simulink model "demo3_model"  (R2024b)
settings: Solver=FixedStepAuto  StartTime=0.0  StopTime=5/60  FixedStep=1/12000  RelTol=1e-3
InitFcn:
  | Vdc1= 35;
  | Vdc2= 35;
  | Vdc3= 35;
  | Vdc4= 35;
  | Vdc5= 35;
  | 
  | GA_th = [58    21    17    49    14];
undefined symbols (not defined in the file): Vdc
libraries: spsDCVoltageSourceLib x5, spsFullBridgeConverterLib x5, spsVoltageMeasurementLib x5, spsSeriesRLCBranchLib x1, simulink x1, spspowerguiLib x1
settings Model: Creator=pgm
settings SolverCC: AlgebraicLoopSolver=TrustRegion
settings DataIOCC: ReturnWorkspaceOutputs=off
settings ModelReferenceCC: EnableRefExpFcnMdlSchedulingChecks=on
settings RTWCC: GPUComputeCapability=3.5

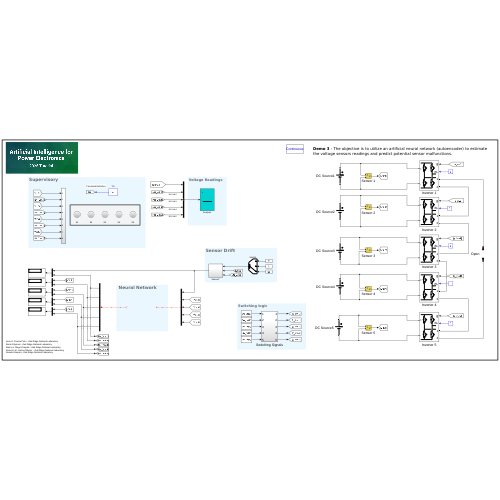
[thumbnail: Simulink's stored preview of the top-level diagram]
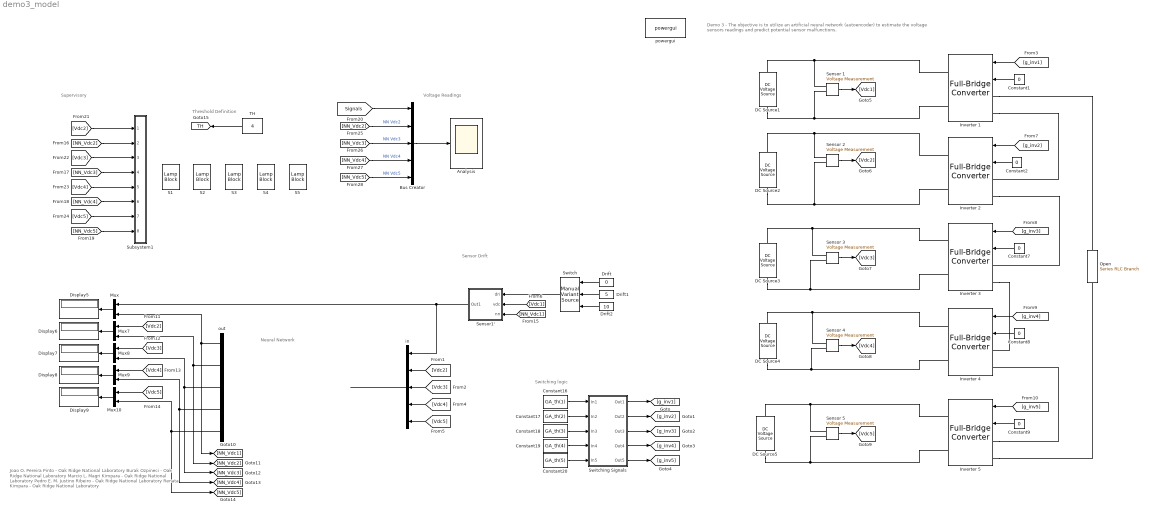
== system demo3_model ==
  note: Threshold Definition
  note: Switching logic
  note: Demo 3 - The objective is to utilize an artificial neural network (autoencoder) to estimate the voltage sensors readings and predict potential sensor malfunctions.
  note: Neural Network
  note: Sensor Drift
  note: Supervisory
  note: Voltage Readings
  note: Joao O. Pereira Pinto - Oak Ridge National Laboratory
      | Burak Ozpineci - Oak Ridge National Laboratory
      | Marcio L. Magri Kimpara - Oak Ridge National Laboratory
      | Pedro E. M. Justino Ribeiro - Oak Ridge National Laboratory
      | Renata Kimpara - Oak Ridge National Laboratory
  Analysis : Scope
  Bus Creator : BusCreator  Inputs=5
  Constant{1..2,7..9} (5 alike) : Constant  Value=0
  Constant16 : Constant  Value=GA_th(1)
  Constant17 : Constant  Value=GA_th(2)
  Constant18 : Constant  Value=GA_th(3)
  Constant19 : Constant  Value=GA_th(4)
  Constant20 : Constant  Value=GA_th(5)
  DC Source{1..5} (5 alike) : spsDCVoltageSourceLib/DC Voltage Source  Amplitude=Vdc  Measurements=None
  Display{5..9} (5 alike) : Display
  Drift : Constant  Value=0
  Drift1 : Constant  Value=5
  Drift2 : Constant  Value=10
  Inverter {1..5} (5 alike) : spsFullBridgeConverterLib/Full-Bridge Converter  ModelType=Switching devices  Ron=1e-3  Rs=1e6  Cs=inf  Vforward=[0,0]  Ron_Diode=1e-3  Rs_Diode=1e6  Cs_Diode=inf  Vf_Diode=1e-3  Rs_CurrentSource=inf  Ron_ACsource=1e-3
      settings: LibrarySourceBlock=sps_lib/Power Electronics/Full-Bridge Converter
  Mux{,7..10} (5 alike) : Mux  Inputs=2
  Open : spsSeriesRLCBranchLib/Series RLC Branch  LConnTagsString=__new0  RConnTagsString=__new0  BranchType=Open circuit  Resistance=10e3  Inductance=1e-6  SetiL0=off  InitialCurrent=0  Capacitance=400e-6  Setx0=off  InitialVoltage=0  Measurements=None
  S{1..5} (5 alike) : LampBlock  LabelPosition=Hide
  Sensor {1..5} (5 alike) : spsVoltageMeasurementLib/Voltage Measurement  Tag=PoWeRsYsTeMmEaSuReMeNt  PhasorSimulation=off  OutputType=Magnitude  PSBequivalent=0
  Sensor1' : Subsystem
  Subsystem1 : Subsystem
  Switch : simulink/Signal Routing/Manual Variant Source  NumChoices=3  LabelModeActiveChoice=V_3
  Switching Signals : Subsystem
  TH : Constant  Value=4
  in : Mux  Inputs=5
  out : Demux  Outputs=5
  powergui : spspowerguiLib/powergui  Priority=1  SimulationMode=Continuous  SampleTime=1e-6  frequency=60  Iterations=50  frequencyindice=0  Pbase=100e6  ErrMax=1e-4  UnitsV=kV  UnitsW=MW  buscounter=0  FunctionMessages=off  echomessages=off  EnableUseOfTLC=off  CurrentSourceSwitches=off  DisableSnubberDevices=off  DisableRonSwitches=off  DisableVfSwitches=off  DisplayEquations=off  AutomaticDiscreteSolvers=off  SolverType=Tustin/Backward Euler (TBE)  Interpol=off  ExternalGateDelay=off  methode=off  Ts=100  x0status=blocks  SPID=on  SwTol=0  HookPort=off  NonlinearTolerance=1e-4  nMaxIteration=100  ContinueOnMaxIteration=off  RestoreLinks=warning  ResistiveCurrentMeasurement=off  Frange=[0:2:500]  Ylog=off  Xlog=on  ShowGrid=off  save=off  variable=ZData  structure=0  ZoomFFT=off  StartTime=0.0  cycles=1  DisplayStyle=1  fundamental=60  FreqAxis=off  MaxFrequency=1000  frequencyindicesteady=1  RmsSteady=1  display=off
  tag scope: TH=global
  wires:
  Constant1/1 -> Inverter 1/2
  Constant2/1 -> Inverter 2/2
  [g_inv1] -> Inverter 1/1
  [g_inv2] -> Inverter 2/1
  [g_inv4] -> Inverter 4/1
  [g_inv3] -> Inverter 3/1
  Constant8/1 -> Inverter 4/2
  Constant7/1 -> Inverter 3/2
  Constant9/1 -> Inverter 5/2
  [g_inv5] -> Inverter 5/1
  Constant16/1 -> Switching Signals/1(In1)
  Constant17/1 -> Switching Signals/2(In2)
  Constant18/1 -> Switching Signals/3(In3)
  Constant19/1 -> Switching Signals/4(In4)
  Constant20/1 -> Switching Signals/5(In5)
  Switching Signals/1(Out1) -> [g_inv1]
  Switching Signals/2(Out2) -> [g_inv2]
  Switching Signals/3(Out3) -> [g_inv3]
  Switching Signals/4(Out4) -> [g_inv4]
  Switching Signals/5(Out5) -> [g_inv5]
  in/1 -> ?
  ? -> out/1
  Sensor 1/1 -> [Vdc1]
  Sensor 2/1 -> [Vdc2]
  Sensor 5/1 -> [Vdc5]
  Sensor 4/1 -> [Vdc4]
  Sensor 3/1 -> [Vdc3]
  [Vdc2] -> in/2
  [Vdc4] -> in/4
  [Vdc5] -> in/5
  Mux/1 -> Display5/1
  Mux7/1 -> Display6/1
  Mux8/1 -> Display7/1
  Mux9/1 -> Display8/1
  Mux10/1 -> Display9/1
  Switch/1 -> Sensor1'/1(dri)
  [Vdc1] -> Sensor1'/2(vdc)
  [Vdc2] -> Mux7/1
  [Vdc3] -> Mux8/1
  [Vdc4] -> Mux9/1
  [Vdc5] -> Mux10/1
  out/1 -> Mux/2, [NN_Vdc1]
  out/2 -> Mux7/2, [NN_Vdc2]
  out/3 -> [NN_Vdc3], Mux8/2
  out/4 -> [NN_Vdc4], Mux9/2
  out/5 -> [NN_Vdc5], Mux10/2
  [NN_Vdc1] -> Sensor1'/3(nn)
  [Vdc3] -> in/3
  [Signals] -> Bus Creator/1
  [NN_Vdc2] -> Bus Creator/2  "NN Vdc2"
  [NN_Vdc3] -> Bus Creator/3  "NN Vdc3"
  [NN_Vdc4] -> Bus Creator/4  "NN Vdc4"
  [NN_Vdc5] -> Bus Creator/5  "NN Vdc5"
  Bus Creator/1 -> Analysis/1
  Drift2/1 -> Switch/3
  [NN_Vdc5] -> Subsystem1/8(In10)
  [Vdc2] -> Subsystem1/1(In3)
  [NN_Vdc4] -> Subsystem1/6(In8)
  [Vdc5] -> Subsystem1/7(In9)
  [Vdc4] -> Subsystem1/5(In7)
  [Vdc3] -> Subsystem1/3(In5)
  [NN_Vdc2] -> Subsystem1/2(In4)
  [NN_Vdc3] -> Subsystem1/4(In6)
  Drift/1 -> Switch/1
  Drift1/1 -> Switch/2
  TH/1 -> [TH]
  Sensor1'/1(Out1) -> Mux/1, in/1
  connections:
  Sensor 1/LConn1 -- DC Source1/RConn1 -- Inverter 1/RConn1
  Sensor 1/LConn2 -- DC Source1/LConn1 -- Inverter 1/RConn2
  Inverter 2/RConn1 -- DC Source2/RConn1 -- Sensor 2/LConn1
  Sensor 2/LConn2 -- DC Source2/LConn1 -- Inverter 2/RConn2
  Inverter 5/LConn2 -- Open/RConn1
  Inverter 1/LConn1 -- Open/LConn1
  Sensor 4/LConn1 -- DC Source4/RConn1 -- Inverter 4/RConn1
  DC Source3/LConn1 -- Sensor 3/LConn2 -- Inverter 3/RConn2
  Sensor 4/LConn2 -- DC Source4/LConn1 -- Inverter 4/RConn2
  DC Source3/RConn1 -- Sensor 3/LConn1 -- Inverter 3/RConn1
  Sensor 5/LConn2 -- DC Source5/LConn1 -- Inverter 5/RConn2
  Sensor 5/LConn1 -- DC Source5/RConn1 -- Inverter 5/RConn1
  Inverter 1/LConn2 -- Inverter 2/LConn1
  Inverter 2/LConn2 -- Inverter 3/LConn1
  Inverter 3/LConn2 -- Inverter 4/LConn1
  Inverter 5/LConn1 -- Inverter 4/LConn2

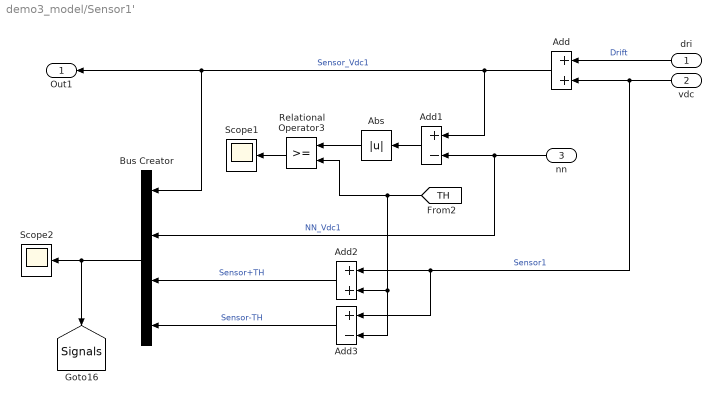
== system demo3_model/Sensor1' ==
  dri : Inport
  vdc : Inport  Port=2
  nn : Inport  Port=3
  Abs : Abs  SaturateOnIntegerOverflow=off
  Add : Sum
  Add1 : Sum  Inputs=+-
  Add2 : Sum
  Add3 : Sum  Inputs=+-
  Bus Creator : BusCreator  Inputs=4
  Relational Operator3 : RelationalOperator  OutDataTypeStr=boolean  RndMeth=Simplest  InputSameDT=off
  Scope1 : Scope
  Scope2 : Scope
  Out1 : Outport
  tag scope: Signals=global
  wires:
  Add/1 -> Out1/1, Bus Creator/1, Add1/1  "Sensor_Vdc1"
  nn/1 -> Bus Creator/2, Add1/2  "NN_Vdc1"
  [TH] -> Add3/2, Add2/2, Relational Operator3/2
  Add1/1 -> Abs/1
  Abs/1 -> Relational Operator3/1
  Relational Operator3/1 -> Scope1/1
  dri/1 -> Add/1  "Drift"
  vdc/1 -> Add3/1, Add2/1, Add/2  "Sensor1"
  Add2/1 -> Bus Creator/3  "Sensor+TH"
  Add3/1 -> Bus Creator/4  "Sensor-TH"
  Bus Creator/1 -> [Signals], Scope2/1

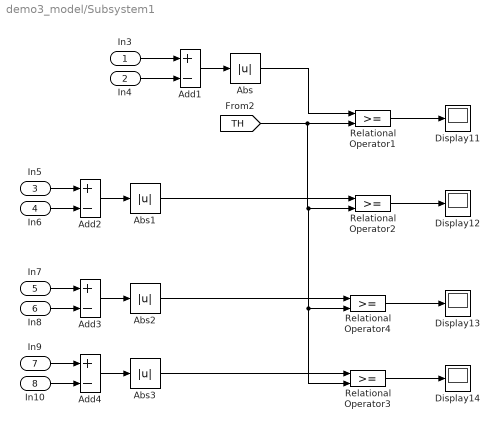
== system demo3_model/Subsystem1 ==
  In3 : Inport
  In4 : Inport  Port=2
  In5 : Inport  Port=3
  In6 : Inport  Port=4
  In7 : Inport  Port=5
  In8 : Inport  Port=6
  In9 : Inport  Port=7
  In10 : Inport  Port=8
  Abs{,1..3} (4 alike) : Abs  SaturateOnIntegerOverflow=off
  Add{1..4} (4 alike) : Sum  Inputs=+-
  Display{11..14} (4 alike) : Display
  Relational Operator{1..4} (4 alike) : RelationalOperator  OutDataTypeStr=boolean  RndMeth=Simplest  InputSameDT=off
  wires:
  Relational Operator3/1 -> Display14/1
  Relational Operator4/1 -> Display13/1
  Relational Operator1/1 -> Display11/1
  Relational Operator2/1 -> Display12/1
  Add1/1 -> Abs/1
  In3/1 -> Add1/1
  In4/1 -> Add1/2
  Abs/1 -> Relational Operator1/1
  [TH] -> Relational Operator3/2, Relational Operator4/2, Relational Operator2/2, Relational Operator1/2
  Add2/1 -> Abs1/1
  In5/1 -> Add2/1
  In6/1 -> Add2/2
  Abs1/1 -> Relational Operator2/1
  Add3/1 -> Abs2/1
  In7/1 -> Add3/1
  In8/1 -> Add3/2
  Abs2/1 -> Relational Operator4/1
  In9/1 -> Add4/1
  In10/1 -> Add4/2
  Add4/1 -> Abs3/1
  Abs3/1 -> Relational Operator3/1

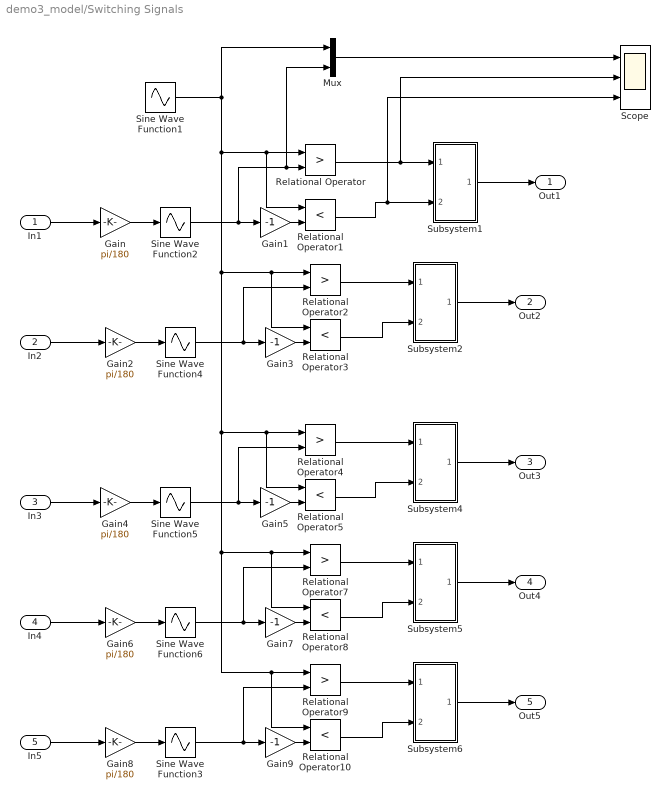
== system demo3_model/Switching Signals ==
  In1 : Inport
  In2 : Inport  Port=2
  In3 : Inport  Port=3
  In4 : Inport  Port=4
  In5 : Inport  Port=5
  Gain{,2,4,6,8} (5 alike) : Gain  Gain=pi/180
  Gain{1,3,5,7,9} (5 alike) : Gain  Gain=-1
  Mux : Mux  Inputs=2
  Relational Operator{,2,4,7,9} (5 alike) : RelationalOperator  Operator=>  OutDataTypeStr=boolean  RndMeth=Simplest  InputSameDT=off
  Relational Operator{1,3,5,8,10} (5 alike) : RelationalOperator  Operator=<  OutDataTypeStr=boolean  RndMeth=Simplest  InputSameDT=off
  Scope : Scope  NumInputPorts=3
  Sine Wave Function1 : Sin  Frequency=2*pi*60  SampleTime=0
  Sine Wave Function{2..6} (5 alike) : Sin  TimeSource=Use external signal  SampleTime=0
  Subsystem1 : Subsystem
  Subsystem2 : Subsystem
  Subsystem4 : Subsystem
  Subsystem5 : Subsystem
  Subsystem6 : Subsystem
  Out1 : Outport
  Out2 : Outport  Port=2
  Out3 : Outport  Port=3
  Out4 : Outport  Port=4
  Out5 : Outport  Port=5
  wires:
  Gain3/1 -> Relational Operator3/2
  Relational Operator10/1 -> Subsystem6/2(In1)
  Sine Wave Function1/1 -> Mux/1, Relational Operator4/1, Relational Operator5/1, Relational Operator9/1, Relational Operator10/1, Relational Operator8/1, Relational Operator7/1, Relational Operator2/1, Relational Operator3/1, Relational Operator1/1, Relational Operator/1
  Relational Operator9/1 -> Subsystem6/1(In2)
  Relational Operator/1 -> Scope/2, Subsystem1/1(In2)
  Relational Operator8/1 -> Subsystem5/2(In1)
  Sine Wave Function4/1 -> Relational Operator2/2, Gain3/1
  Gain5/1 -> Relational Operator5/2
  Sine Wave Function2/1 -> Gain1/1, Mux/2, Relational Operator/2
  Gain1/1 -> Relational Operator1/2
  In4/1 -> Gain6/1
  Gain/1 -> Sine Wave Function2/1
  Sine Wave Function3/1 -> Relational Operator9/2, Gain9/1
  Subsystem6/1(Out1) -> Out5/1
  Relational Operator5/1 -> Subsystem4/2(In1)
  Sine Wave Function6/1 -> Gain7/1, Relational Operator7/2
  Gain2/1 -> Sine Wave Function4/1
  Gain9/1 -> Relational Operator10/2
  Sine Wave Function5/1 -> Relational Operator4/2, Gain5/1
  Subsystem4/1(Out1) -> Out3/1
  Gain7/1 -> Relational Operator8/2
  Gain8/1 -> Sine Wave Function3/1
  Gain4/1 -> Sine Wave Function5/1
  Relational Operator1/1 -> Scope/3, Subsystem1/2(In1)
  Relational Operator4/1 -> Subsystem4/1(In2)
  Subsystem2/1(Out1) -> Out2/1
  Relational Operator7/1 -> Subsystem5/1(In2)
  Gain6/1 -> Sine Wave Function6/1
  Relational Operator3/1 -> Subsystem2/2(In1)
  In2/1 -> Gain2/1
  In5/1 -> Gain8/1
  Relational Operator2/1 -> Subsystem2/1(In2)
  Subsystem1/1(Out1) -> Out1/1
  In1/1 -> Gain/1
  In3/1 -> Gain4/1
  Subsystem5/1(Out1) -> Out4/1
  Mux/1 -> Scope/1

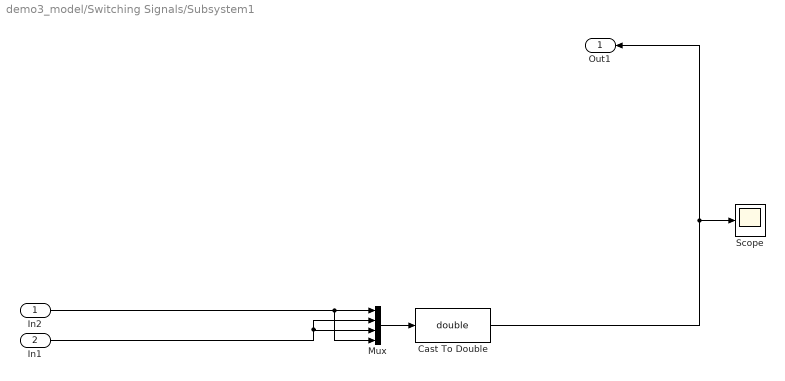
== system demo3_model/Switching Signals/Subsystem1 ==
  In2 : Inport
  In1 : Inport  Port=2
  Cast To Double : DataTypeConversion  OutDataTypeStr=double  SaturateOnIntegerOverflow=off  RndMeth=Floor
  Mux : Mux
  Scope : Scope
  Out1 : Outport
  wires:
  Cast To Double/1 -> Scope/1, Out1/1
  In2/1 -> Mux/4, Mux/1
  In1/1 -> Mux/3, Mux/2
  Mux/1 -> Cast To Double/1

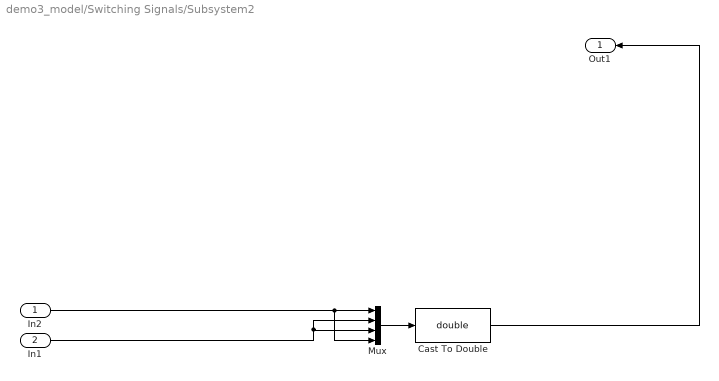
== system demo3_model/Switching Signals/Subsystem2 ==
  In2 : Inport
  In1 : Inport  Port=2
  Cast To Double : DataTypeConversion  OutDataTypeStr=double  SaturateOnIntegerOverflow=off  RndMeth=Floor
  Mux : Mux
  Out1 : Outport
  wires:
  Mux/1 -> Cast To Double/1
  In1/1 -> Mux/2, Mux/3
  In2/1 -> Mux/1, Mux/4
  Cast To Double/1 -> Out1/1

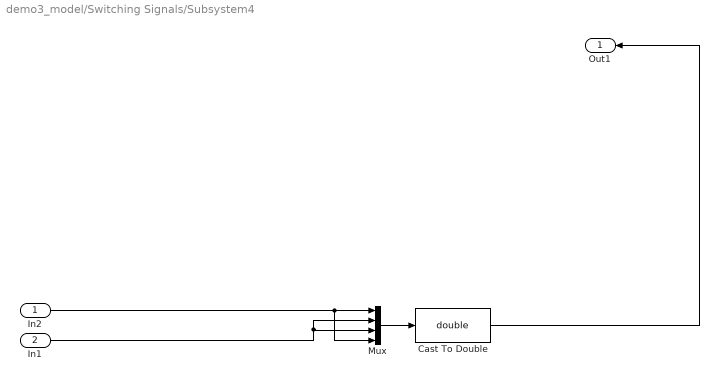
== system demo3_model/Switching Signals/Subsystem4 ==
  In2 : Inport
  In1 : Inport  Port=2
  Cast To Double : DataTypeConversion  OutDataTypeStr=double  SaturateOnIntegerOverflow=off  RndMeth=Floor
  Mux : Mux
  Out1 : Outport
  wires:
  Cast To Double/1 -> Out1/1
  In2/1 -> Mux/4, Mux/1
  In1/1 -> Mux/3, Mux/2
  Mux/1 -> Cast To Double/1

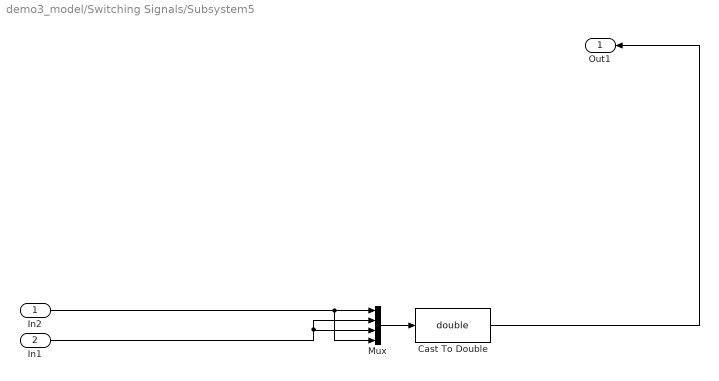
== system demo3_model/Switching Signals/Subsystem5 ==
  In2 : Inport
  In1 : Inport  Port=2
  Cast To Double : DataTypeConversion  OutDataTypeStr=double  SaturateOnIntegerOverflow=off  RndMeth=Floor
  Mux : Mux
  Out1 : Outport
  wires:
  Mux/1 -> Cast To Double/1
  In1/1 -> Mux/2, Mux/3
  In2/1 -> Mux/1, Mux/4
  Cast To Double/1 -> Out1/1

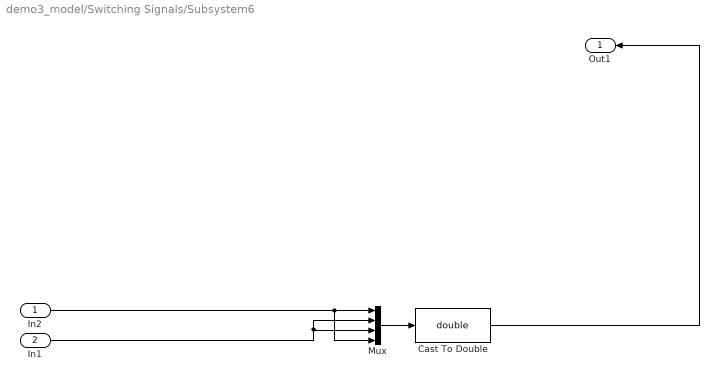
== system demo3_model/Switching Signals/Subsystem6 ==
  In2 : Inport
  In1 : Inport  Port=2
  Cast To Double : DataTypeConversion  OutDataTypeStr=double  SaturateOnIntegerOverflow=off  RndMeth=Floor
  Mux : Mux
  Out1 : Outport
  wires:
  Cast To Double/1 -> Out1/1
  In2/1 -> Mux/4, Mux/1
  In1/1 -> Mux/3, Mux/2
  Mux/1 -> Cast To Double/1
